simulink model "Active_Suspension_Simulink_Model"  (R2023a)
settings: Solver=ode23tb  StartTime=0.0  StopTime=10  RelTol=1e-3
model workspace (MAT data in the model file):
  Ks = 16000
  Kt = 190000
  Mb = 300
  Mw = 60
  bs = 1000
  mb = 300
  mw = 60
settings Model: Creator=poke  LastModifiedBy=poke
settings OptimizationCC: ReuseModelBlockBuffer=off

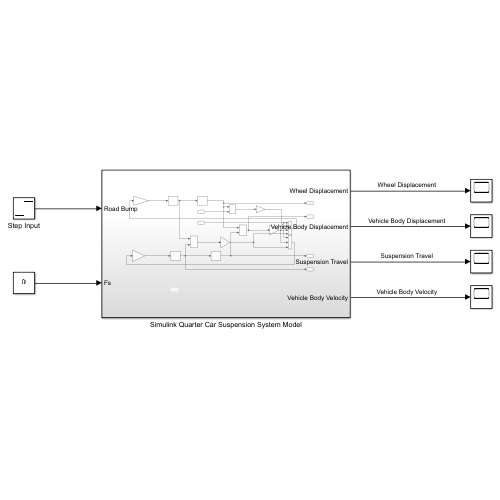
[thumbnail: Simulink's stored preview of the top-level diagram]
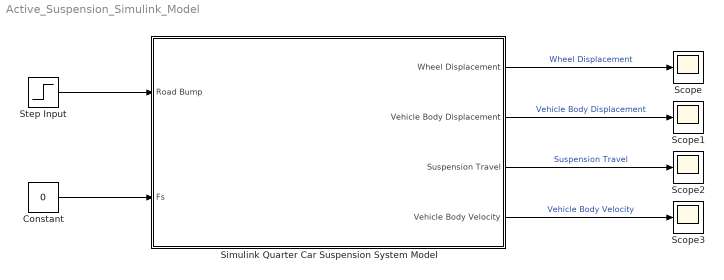
== system Active_Suspension_Simulink_Model ==
  Constant : Constant  Value=0
  Scope{,1..3} (4 alike) : Scope
  Simulink Quarter Car Suspension System Model : Subsystem
  Step Input : Step  SampleTime=0
  wires:
  Simulink Quarter Car Suspension System Model/1(Wheel Displacement) -> Scope/1  "Wheel Displacement"
  Simulink Quarter Car Suspension System Model/2(Vehicle Body Displacement) -> Scope1/1  "Vehicle Body Displacement"
  Simulink Quarter Car Suspension System Model/3(Suspension Travel) -> Scope2/1  "Suspension Travel"
  Simulink Quarter Car Suspension System Model/4(Vehicle Body Velocity) -> Scope3/1  "Vehicle Body Velocity"
  Constant/1 -> Simulink Quarter Car Suspension System Model/2(Fs)
  Step Input/1 -> Simulink Quarter Car Suspension System Model/1(Road Bump)

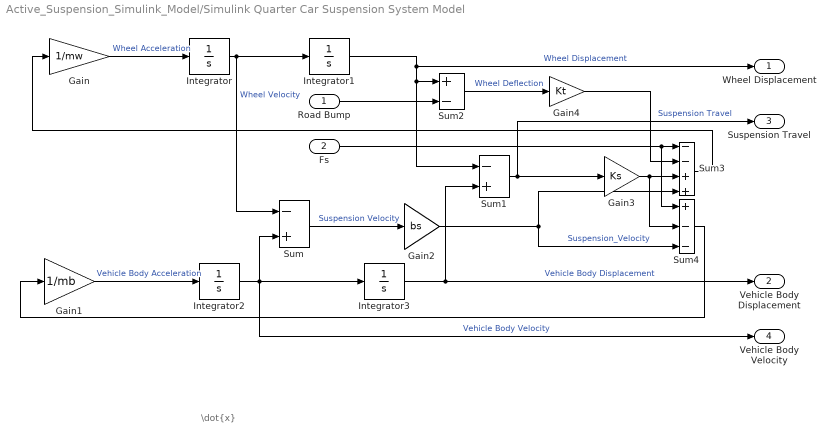
== system Active_Suspension_Simulink_Model/Simulink Quarter Car Suspension System Model ==
  note: \dot{x}
  Road Bump : Inport
  Fs : Inport  Port=2
  Gain : Gain  Gain=1/mw
  Gain1 : Gain  Gain=1/mb
  Gain2 : Gain  Gain=bs
  Gain3 : Gain  Gain=Ks
  Gain4 : Gain  Gain=Kt
  Integrator{,1..3} (4 alike) : Integrator
  Sum : Sum  Inputs=-+
  Sum1 : Sum  Inputs=-+
  Sum2 : Sum  Inputs=+-
  Sum3 : Sum  Inputs=--++
  Sum4 : Sum  Inputs=+--
  Wheel Displacement : Outport
  Vehicle Body Displacement : Outport  Port=2
  Suspension Travel : Outport  Port=3
  Vehicle Body Velocity : Outport  Port=4
  wires:
  Gain/1 -> Integrator/1  "Wheel Acceleration"
  Gain2/1 -> Sum3/4, Sum4/3  "Suspension_Velocity"
  Sum4/1 -> Gain1/1
  Gain1/1 -> Integrator2/1  "Vehicle Body Acceleration"
  Sum2/1 -> Gain4/1  "Wheel Deflection"
  Sum3/1 -> Gain/1
  Sum/1 -> Gain2/1  "Suspension Velocity"
  Integrator2/1 -> Sum/2, Vehicle Body Velocity/1, Integrator3/1  "Vehicle Body Velocity"
  Integrator1/1 -> Wheel Displacement/1, Sum2/1, Sum1/1  "Wheel Displacement"
  Integrator3/1 -> Vehicle Body Displacement/1, Sum1/2  "Vehicle Body Displacement"
  Integrator/1 -> Integrator1/1, Sum/1  "Wheel Velocity"
  Gain3/1 -> Sum3/3, Sum4/2
  Road Bump/1 -> Sum2/2
  Sum1/1 -> Gain3/1, Suspension Travel/1  "Suspension Travel"
  Gain4/1 -> Sum3/2
  Fs/1 -> Sum3/1, Sum4/1
